simulink model "STR_Test_Template_2024_Abgabe"  (R2024a)
settings: Solver=FixedStepDiscrete  StartTime=0.0  StopTime=inf  FixedStep=.01  RelTol=1e-3  EnableMultiTasking=on
libraries: simulink x5
Description:
  | Provides a STR algorithm with variable
  | control structure, depending on the zeros of Zc
  | 
  | Order to switch on:
  | 1. Estimater
  | 2. Design
  | 3. Controller
settings Model: Creator=jreuter  LastModifiedBy=danie
settings SolverCC: AlgebraicLoopSolver=TrustRegion
settings DataIOCC: LimitDataPoints=on  SaveFormat=Array  SignalLoggingSaveFormat=ModelDataLogs  ReturnWorkspaceOutputs=off
settings OptimizationCC: BlockReduction=off  OptimizeBlockIOStorage=off  BufferReuse=off  GlobalBufferReuse=off  ExpressionFolding=off  ExpressionDepthLimit=2147483647  LocalBlockOutputs=off  LifeSpan=inf
settings DebuggingCC: UnderspecifiedInitializationDetection=Classic  MergeDetectMultiDrivingBlocksExec=none  SolverPrmCheckMsg=warning  FcnCallInpInsideContextMsg=warning  UnconnectedInputMsg=warning  UnconnectedOutputMsg=warning  UnconnectedLineMsg=warning  StateNameClashWarn=warning  SFUnexpectedBacktrackingDiag=warning  SFNoUnconditionalDefaultTransitionDiag=warning  SFExecutionAtInitializationDiag=none  ArithmeticOperatorsInVariantConditions=warning
settings HardwareCC: ProdBitPerPointer=32  ProdBitPerSizeT=32  ProdBitPerPtrDiffT=32  ProdLargestAtomicFloat=None  ProdIntDivRoundTo=Undefined  ProdEndianess=Unspecified  ProdWordSize=32  ProdHWDeviceType=32-bit Generic
settings ModelReferenceCC: EnableRefExpFcnMdlSchedulingChecks=on  PropagateSignalLabelsOutOfModel=off
settings SFSimCC: SimUseLocalCustomCode=off  CustomCodeUndefinedFunction=UseInterfaceOnly
settings RTWCC: Description=Generic Real-Time Target with dynamic memory allocation  SystemTargetFile=grt_malloc.tlc  TemplateMakefile=grt_malloc_default_tmf  GenerateReport=on  RTWUseLocalCustomCode=off  LaunchReport=on  GPUComputeCapability=3.5  DLArmComputeVersion=19.05
settings CodeAppCC: StateflowObjectComments=on
settings GRTTargetCC: TargetLangStandard=C89/C90 (ANSI)  CombineOutputUpdateFcns=off  GRTInterface=on  UseMalloc=on  ExtModeMexFile=noextcomm
settings ConfigComp: CovMetricSettings=dw  CovSaveCumulativeToWorkspaceVar=on  CovSaveSingleToWorkspaceVar=on  CovExternalEMLEnable=off

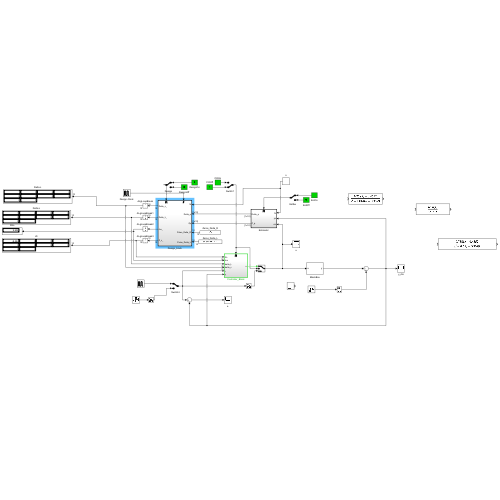
[thumbnail: Simulink's stored preview of the top-level diagram]
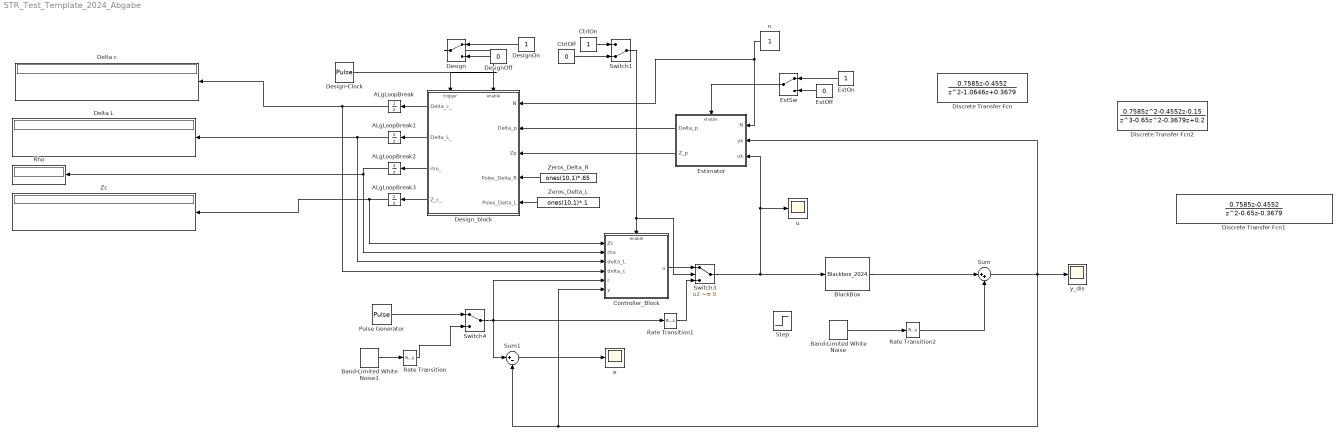
== system STR_Test_Template_2024_Abgabe ==
  ALgLoopBreak{,1..3} (4 alike) : UnitDelay  SampleTime=-1  HasFrameUpgradeWarning=on
  Band-Limited White Noise : simulink/Sources/Band-Limited White Noise  Cov=[1e-6]  Ts=.01  seed=[23341]
  Band-Limited White Noise1 : simulink/Sources/Band-Limited White Noise  Cov=[0.5]  Ts=.05  seed=[23341]
  BlackBox : S-Function  FunctionName=Blackbox_2024  SFunctionDeploymentMode=off  EnableBusSupport=off
      mask Display:
      | port_label('input',1,'u')
      | port_label('output',1,'y')
  Controller_Block : Subsystem
  CtrlOff : Constant  Value=0  SampleTime=-1
  CtrlOn : Constant  SampleTime=-1
  Delta L : Display
  Delta c : Display
  Design : ManualSwitch
  Design-Clock : DiscretePulseGenerator  PulseType=Time based  Period=.5  PulseWidth=50
  DesignOff : Constant  Value=0  SampleTime=-1
  DesignOn : Constant  SampleTime=-1
  Design_block : Subsystem
  Discrete Transfer Fcn : DiscreteTransferFcn  Numerator=[0.7585 -0.4552]  Denominator=[1 -1.0646 0.3679]
  Discrete Transfer Fcn1 : DiscreteTransferFcn  Numerator=[0.7585 -0.4552]  Denominator=[1 -0.65 -0.3679]
  Discrete Transfer Fcn2 : DiscreteTransferFcn  Numerator=[0.7585 -0.4552 -0.15]  Denominator=[1 -0.65 -0.3679 0.2]
  EstOff : Constant  Value=0  SampleTime=-1
  EstOn : Constant  SampleTime=-1
  EstSw : ManualSwitch
  Estimator : Subsystem
  Pulse Generator : DiscretePulseGenerator  PulseType=Time based  Period=1  PulseWidth=50
  Rate Transition : RateTransition  Integrity=off  OutPortSampleTimeOpt=Inherit
  Rate Transition1 : RateTransition  Integrity=off  OutPortSampleTimeOpt=Inherit
  Rate Transition2 : RateTransition  Integrity=off  OutPortSampleTimeOpt=Inherit
  Rho : Display
  Step : Step  SampleTime=0
  Sum : Sum  Inputs=|++
  Sum1 : Sum  Inputs=|+-
  Switch1 : ManualSwitch  CurrentSetting=0
  Switch3 : Switch  Criteria=u2 ~= 0  SaturateOnIntegerOverflow=off  InputSameDT=off
  Switch4 : ManualSwitch
  Zc : Display
  Zeros_Delta_L : Constant  Value=ones(10,1)*.1
  Zeros_Delta_R : Constant  Value=ones(10,1)*.65
  e : Scope
  n : Constant
  u : Scope
  y_dis : Scope
  wires:
  Band-Limited White Noise1/1 -> Rate Transition/1
  Sum/1 -> y_dis/1, Estimator/2(yk), Controller_Block/6(y), Sum1/2
  n/1 -> Estimator/1(N), Design_block/1(N)
  EstOff/1 -> EstSw/2
  EstOn/1 -> EstSw/1
  Switch1/1 -> Controller_Block/Enable, Switch3/2
  CtrlOff/1 -> Switch1/2
  CtrlOn/1 -> Switch1/1
  Estimator/1(Delta_p) -> Design_block/2(Delta_p)
  Estimator/2(Z_p) -> Design_block/3(Zp)
  Zeros_Delta_R/1 -> Design_block/4(Poles_Delta_R)
  Zeros_Delta_L/1 -> Design_block/5(Poles_Delta_L)
  Band-Limited White Noise/1 -> Rate Transition2/1
  Switch4/1 -> Rate Transition1/1, Controller_Block/5(r), Sum1/1
  Pulse Generator/1 -> Switch4/1
  Controller_Block/1(u) -> Switch3/1
  Rate Transition/1 -> Switch4/2
  Rate Transition1/1 -> Switch3/3
  Switch3/1 -> BlackBox/1, u/1, Estimator/3(uk)
  Sum1/1 -> e/1
  Design_block/4(Z_c_) -> ALgLoopBreak3/1
  Design_block/1(Delta_c_) -> ALgLoopBreak/1
  Design_block/3(rho_) -> ALgLoopBreak2/1
  Design_block/2(Delta_L_) -> ALgLoopBreak1/1
  EstSw/1 -> Estimator/Enable
  DesignOff/1 -> Design/2
  DesignOn/1 -> Design/1
  Design/1 -> Design_block/Enable
  Design-Clock/1 -> Design_block/Trigger
  ALgLoopBreak1/1 -> Delta L/1, Controller_Block/3(delta_L)
  ALgLoopBreak/1 -> Delta c/1, Controller_Block/4(delta_c)
  ALgLoopBreak3/1 -> Controller_Block/1(Zc), Zc/1
  ALgLoopBreak2/1 -> Rho/1, Controller_Block/2(rho)
  BlackBox/1 -> Sum/1
  Rate Transition2/1 -> Sum/2

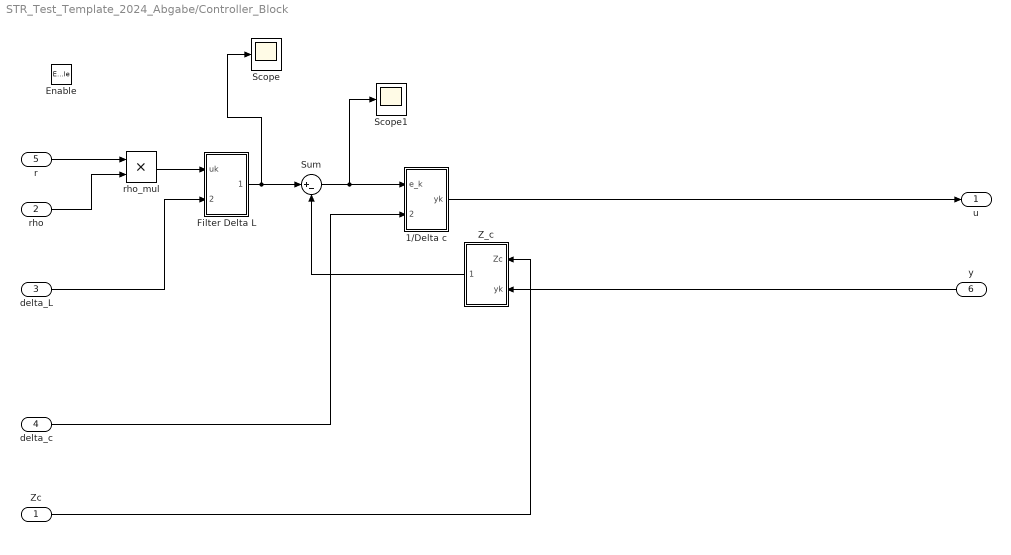
== system STR_Test_Template_2024_Abgabe/Controller_Block ==
  Zc : Inport
  rho : Inport  Port=2
  delta_L : Inport  Port=3
  delta_c : Inport  Port=4
  r : Inport  Port=5
  y : Inport  Port=6
  Enable : EnablePort  StatesWhenEnabling=reset
  1/Delta c : Subsystem
  Filter Delta L : Subsystem
  Scope : Scope
  Scope1 : Scope
  Sum : Sum  Inputs=|+-
  Z_c : Subsystem
  rho_mul : Product  RndMeth=Zero
  u : Outport
  wires:
  r/1 -> rho_mul/1
  delta_c/1 -> 1/Delta c/2(Delta_c)
  rho/1 -> rho_mul/2
  y/1 -> Z_c/2(yk)
  Sum/1 -> Scope1/1, 1/Delta c/1(e_k)
  Z_c/1(u_star) -> Sum/2
  Zc/1 -> Z_c/1(Zc)
  Filter Delta L/1(r_filtered) -> Scope/1, Sum/1
  delta_L/1 -> Filter Delta L/2(Delta_L)
  rho_mul/1 -> Filter Delta L/1(uk)
  1/Delta c/1(yk) -> u/1

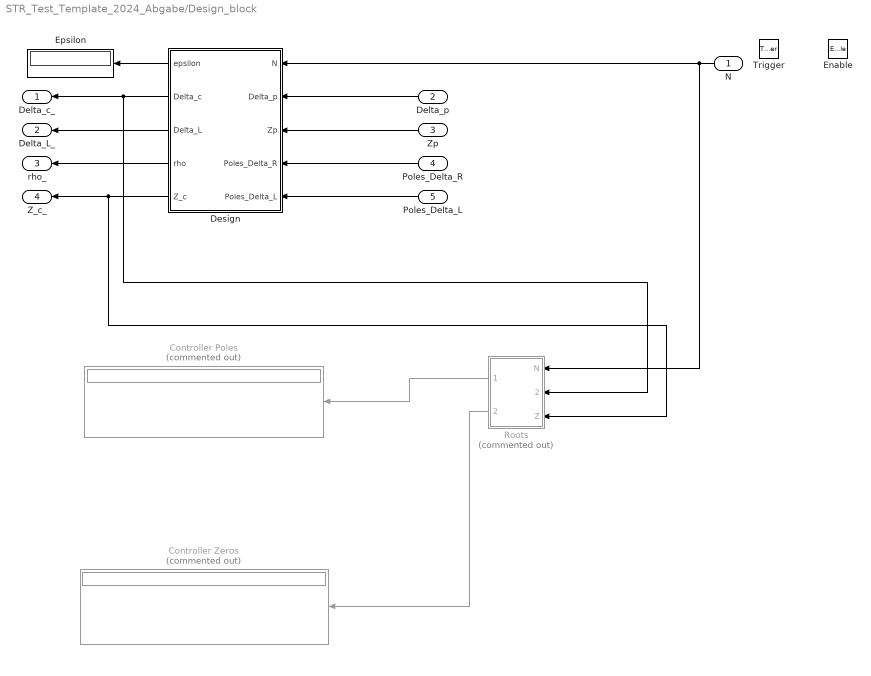
== system STR_Test_Template_2024_Abgabe/Design_block ==
  N : Inport
  Delta_p : Inport  Port=2
  Zp : Inport  Port=3
  Poles_Delta_R : Inport  Port=4
  Poles_Delta_L : Inport  Port=5
  Enable : EnablePort  StatesWhenEnabling=reset
  Trigger : TriggerPort  VariantControl=(inherit)  PortDimensions=1
  Controller Poles : Display  Commented=on
  Controller Zeros : Display  Commented=on
  Design : MATLAB Function  TreatAsAtomicUnit=on
  Epsilon : Display
  Roots : MATLAB Function  Commented=on  TreatAsAtomicUnit=on
  Delta_c_ : Outport
  Delta_L_ : Outport  Port=2
  rho_ : Outport  Port=3
  Z_c_ : Outport  Port=4
  wires:
  Design/1(epsilon) -> Epsilon/1
  N/1 -> Design/1(N), Roots/1(N)
  Delta_p/1 -> Design/2(Delta_p)
  Design/2(Delta_c) -> Delta_c_/1, Roots/2(Delta)
  Zp/1 -> Design/3(Zp)
  Design/3(Delta_L) -> Delta_L_/1
  Poles_Delta_R/1 -> Design/4(Poles_Delta_R)
  Design/4(rho) -> rho_/1
  Poles_Delta_L/1 -> Design/5(Poles_Delta_L)
  Design/5(Z_c) -> Z_c_/1, Roots/3(Z)
  Roots/1(Poles) -> Controller Poles/1
  Roots/2(Zeros) -> Controller Zeros/1

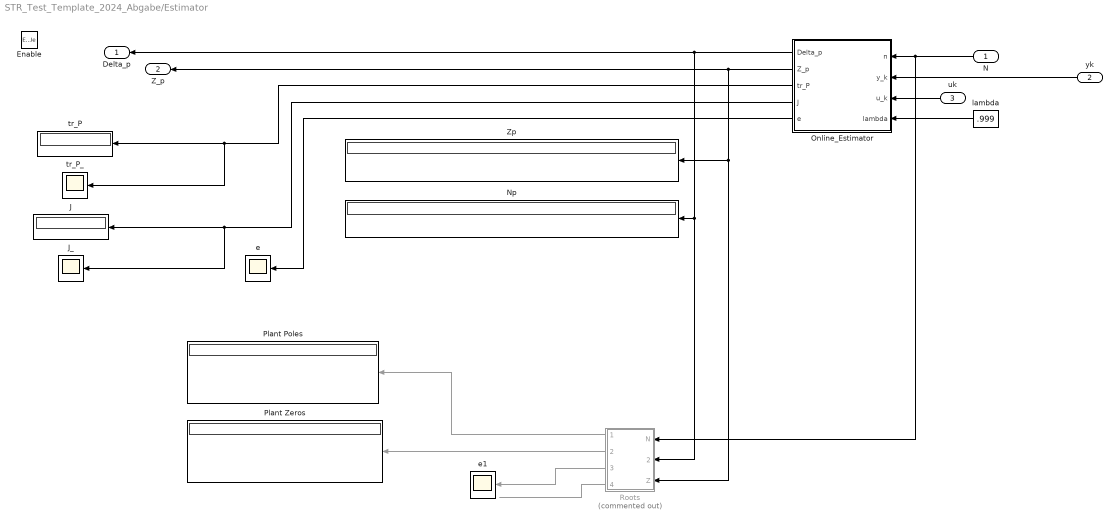
== system STR_Test_Template_2024_Abgabe/Estimator ==
  N : Inport
  yk : Inport  Port=2
  uk : Inport  Port=3
  Enable : EnablePort  StatesWhenEnabling=reset
  J : Display
  J_ : Scope
  Np : Display
  Online_Estimator : MATLAB Function  TreatAsAtomicUnit=on
  Plant Poles : Display
  Plant Zeros : Display
  Roots : MATLAB Function  Commented=on  TreatAsAtomicUnit=on
  Zp : Display
  e : Scope
  e1 : Scope
  lambda : Constant  Value=.999
  tr_P : Display
  tr_P_ : Scope
  Delta_p : Outport
  Z_p : Outport  Port=2
  wires:
  Online_Estimator/4(J) -> J_/1, J/1
  Online_Estimator/5(e) -> e/1
  Online_Estimator/3(tr_P) -> tr_P_/1, tr_P/1
  Online_Estimator/2(Z_p) -> Z_p/1, Roots/3(Z), Zp/1
  Online_Estimator/1(Delta_p) -> Roots/2(Delta), Np/1, Delta_p/1
  uk/1 -> Online_Estimator/3(u_k)
  yk/1 -> Online_Estimator/2(y_k)
  N/1 -> Roots/1(N), Online_Estimator/1(n)
  lambda/1 -> Online_Estimator/4(lambda)
  Roots/1(Poles) -> Plant Poles/1
  Roots/2(Zeros) -> Plant Zeros/1
  Roots/3(Re_Poles) -> e1/1
  Roots/4(Im_Poles) -> ?

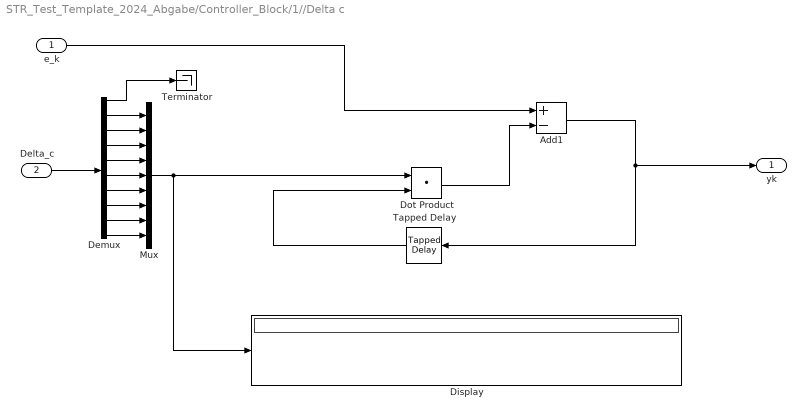
== system STR_Test_Template_2024_Abgabe/Controller_Block/1//Delta c ==
  e_k : Inport
  Delta_c : Inport  Port=2
  Add1 : Sum  Inputs=+-
  Demux : Demux  Outputs=10
  Display : Display
  Dot Product : DotProduct  OutDataTypeStr=Inherit: Inherit via internal rule
  Mux : Mux  Inputs=9
  Tapped Delay : simulink/Discrete/Tapped Delay  vinit=0.0  samptime=-1  NumDelays=9  DelayOrder=Newest  includeCurrent=off
  Terminator : Terminator
  yk : Outport
  wires:
  Tapped Delay/1 -> Dot Product/2
  Add1/1 -> Tapped Delay/1, yk/1
  e_k/1 -> Add1/1
  Dot Product/1 -> Add1/2
  Demux/10 -> Mux/9
  Demux/9 -> Mux/8
  Demux/8 -> Mux/7
  Demux/7 -> Mux/6
  Demux/6 -> Mux/5
  Demux/5 -> Mux/4
  Demux/3 -> Mux/2
  Demux/4 -> Mux/3
  Demux/2 -> Mux/1
  Delta_c/1 -> Demux/1
  Mux/1 -> Display/1, Dot Product/1
  Demux/1 -> Terminator/1

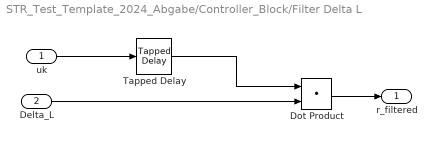
== system STR_Test_Template_2024_Abgabe/Controller_Block/Filter Delta L ==
  uk : Inport
  Delta_L : Inport  Port=2
  Dot Product : DotProduct  OutDataTypeStr=Inherit: Inherit via internal rule
  Tapped Delay : simulink/Discrete/Tapped Delay  vinit=0.0  samptime=-1  NumDelays=9  DelayOrder=Newest  includeCurrent=on
  r_filtered : Outport
  wires:
  Tapped Delay/1 -> Dot Product/1
  Dot Product/1 -> r_filtered/1
  uk/1 -> Tapped Delay/1
  Delta_L/1 -> Dot Product/2

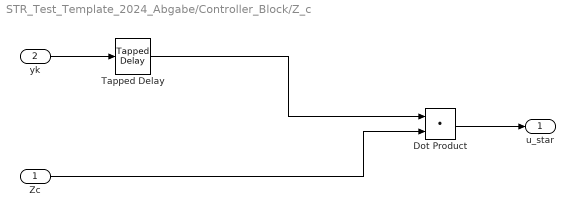
== system STR_Test_Template_2024_Abgabe/Controller_Block/Z_c ==
  Zc : Inport
  yk : Inport  Port=2
  Dot Product : DotProduct  OutDataTypeStr=Inherit: Inherit via internal rule
  Tapped Delay : simulink/Discrete/Tapped Delay  vinit=0.0  samptime=-1  NumDelays=9  DelayOrder=Newest  includeCurrent=on
  u_star : Outport
  wires:
  yk/1 -> Tapped Delay/1
  Zc/1 -> Dot Product/2
  Tapped Delay/1 -> Dot Product/1
  Dot Product/1 -> u_star/1

== matlab function STR_Test_Template_2024_Abgabe/Estimator/Online_Estimator ==
  data: Delta_p output; Z_p output; tr_P output; J output; n input; y_k input; e output; u_k input; lambda input
function [Delta_p, Z_p, tr_P, J, e  ] = fcn(n, y_k, u_k, lambda)
%eml
m = n -1;
persistent P;
persistent theta_hat;
persistent old_n; 
persistent phi;
persistent J_per;
n_max = 10;
Delta_p = zeros(1, n_max);
Z_p = zeros(1, n_max);
ek = 0;


n = min(n, n_max);

if (isempty(old_n))
    old_n = n;
end

%Initialization
if (isempty(P) || old_n ~= n) % If the order variable n has changed -> New initialization
  P = 1e4*eye(2*n_max);
  theta_hat = zeros(2*n_max, 1);
  phi = zeros(2*n_max, 1);
  old_n = n;
  J_per = 0;
end


%Your Code goes here
P = (1/lambda) * (P - ((P*phi*phi'*P)/(phi'*P*phi+lambda))); % Gewichtungsmatrix
K = (P*phi)/(phi'*P*phi+lambda);
e = y_k - phi'*theta_hat;
theta_hat = theta_hat + K*e;

% Extrahieren der vergangenen Ausgangsdaten  
phi(2:n) = phi(1:n-1);
phi(1)   = y_k;
% Extrahieren der vergangenen Eingangsdaten 
phi(n+2:n+m+1) = phi(n+1:n+m);
phi(n+1)   = u_k;
%% Ausgänge
Delta_p(1) = 1;
Delta_p(2:n+1) = theta_hat(1:n);

for i = 2:n+1
    Delta_p(i) = -Delta_p(i);
end
%Delta_p(2:n+1) = Delta_p(2:n+1) * (-1);
Z_p(1:m+1) = theta_hat(n+1:n+m+1);

tr_P = 8;
J = 0.5 * (e^2 + lambda * J_per);
J_per = J;
%J = 0;
%e = 0;

== matlab function STR_Test_Template_2024_Abgabe/Design_block/Design ==
  data: epsilon output; Delta_c output; Delta_L output; N input; Delta_p input; Zp input; rho output; Poles_Delta_R input; Z_c output; Poles_Delta_L input
function [epsilon,Delta_c ,Delta_L, rho, Z_c  ] = fcn(N, Delta_p, Zp, Poles_Delta_R, Poles_Delta_L)
%% Statische Initialisieren 
% Es werden alle Variablen statisch initialisiert um eine 
% dynamische Speicherallokation zu verhindern
n = N;
m = n-1;
max = 10; % Maximale größe

% P initial mit 0 definieren
P = zeros(max,max);
% Initialisieren von lambda und gamma mit max Length
lambda = zeros(1,max); % Initialisieren mit maxLength
gamma  = zeros(1,max); % Initialisieren mit maxLength
% Matrizen für Pseudoinverse vordefinieren
U = zeros(max,max);
S = zeros(max,max);
V = zeros(max,max);

Delta_c = zeros(max,1);
Z_c     = zeros(max,1);
Delta_L = zeros(max,1);

len_deltaP = n+1;
len_Zp     = m+1;

%% Besimmung von n und m und den Koeffizenten von delta_R und delta_L
coeffs_delta_R = poly(Poles_Delta_R(1:n));
coeffs_delta_L = poly(Poles_Delta_L(1:m));

%% Bestimmung der Vektoren Gamma und Lambda
x = conv(coeffs_delta_R, coeffs_delta_L);
gamma(1:length(x)-1) = x(2:end);
gamma = transpose(gamma);
start_index = min(len_deltaP - 1, n); 
lambda(1:start_index) = Delta_p(2:start_index+1);
lambda = transpose(lambda);

%% Erstellung der Matrix P + Invertieren durch Pseudoinverse
P = create_P(Delta_p,Zp,n,m,P,len_Zp,len_deltaP)
% Singulärwertzerlegung (SVD)
[U, S, V] = svd(P);
% Anzahl der Vektoren auswählen
cV = 2*m+1; 
% Pseudoinverse berechnen, indem nur die ersten n Vektoren verwendet werden
Pseudoinverse = V(:, 1:cV) * pinv(S(1:cV, 1:cV)) * U(:, 1:cV)';

%% Berechnen der Koeffizienten durch inv(P) * [gamma - lambda]
coeff = transpose(Pseudoinverse * (gamma-lambda));

%% Bestimmung delta_c, delta_l und Zc  
Delta_c(1)   = 1;
Delta_c(2:m+1) = coeff(1:m); 
Delta_L(1:length(coeffs_delta_L)) = coeffs_delta_L';

Z_c(1:length(coeff)-m)     = coeff(m+1:end); 
%% Bestimme Rho durch Vorgabe von T(1) = 1 mit z = 1

val_delta_c = polyval(flip(Delta_c),1);
val_Zp      = polyval(Zp,1);

%rho = val_Zp / val_delta_c
if val_Zp == 0
    rho = 1;
else
    rho = polyval(coeffs_delta_R,1) / val_Zp;
end    

%rho = 0.5;

%% Bestimmung von epsilon :: TODO
leftSide  = polyval(conv(coeffs_delta_R, coeffs_delta_L),1);
rightSide = polyval(conv(Delta_c,Delta_p),1) + polyval(conv(Zp,Z_c),1);

epsilon = leftSide - rightSide;

end
%% Funktionen 
function P = create_P(Delta_p,Zp,n,m,P, len_Zp, len_deltaP)
    % Erstellung p1_p_delta Dimension (m x m) untere Rechte Dreiecksmatrix
    % (1,1)(1,m)
    % (m,1)(m,m) 
    for i = 1:m
        P(i,1:i) = Delta_p(i:-1:1);
    end
    % Erstellung p2_p_delta Dimension (n x m)
    % (m+1  ,1)(m+1   ,m) 
    % (m+n+1,1)(m+n+1 ,m) 
    % 1. Zeile der Matrix p1 bis p(n-1)
    index = len_deltaP -1;
    for j = 1:m 
        P(m+1,j) = Delta_p(index);
        index = index -1;
    end
    % Obere Rechte Dreieckmatrix erstellen ab Zeile 2
    cStart = 1;
    for i = m+2:2*m+1
        index = len_deltaP;
        for j = cStart:m
            P(i,j) = Delta_p(index);
            index = index - 1;
        end
        cStart = cStart +1;
    end
    % Erstellung p1_c_pi Dimension (n x m)
    % (1 ,m+1)(1 ,2m+2) 
    % (m ,m+1)(m ,2m+2) 
    z = 1;
    count = 0;
    for i = m:-1:1 % Schleife Rückwärtsdurchlaufen
        for j = m+1:2*m+1
            index = len_Zp -z;
            if index <= 0
                break; % Index außerhalb der gültigen Bereichs -> 0 auffüllen
            end
            P(i,j) = Zp(index);
            z = z + 1;
        end
        count = count +1;
        z = 1 + count;
    end
    % Erstellung p2_c_pi Dimension (n x m)
    % (m+1  ,m+1)(m+1 ,2m+1) 
    % (m+n  ,m+1)(m+n ,2m+1)
    for i = m+1:m+n
        index = len_Zp;
        for j = i:2*m+1
            if index > 0
                P(i,j) = Zp(index);
                index = index - 1;
            else
                break; % Da index <= 0, kann die Schleife beenden
            end
        end
    end
end

== matlab function STR_Test_Template_2024_Abgabe/Design_block/Roots ==
  data: Poles output; Zeros output; N input; Delta input; Z input
function [Poles, Zeros  ] = fcn(N, Delta, Z)
%eml 

n_max = 10;
Poles= 1i*zeros(n_max,1);
Zeros = 1i*zeros(n_max,1);


n = min(N, n_max);
% Convert roots to coefs
Poles(1:n-1) = roots(Delta(1:n));
Zeros(1:n-1) = roots(Z(1:n));

== matlab function STR_Test_Template_2024_Abgabe/Estimator/Roots ==
  data: Poles output; Zeros output; N input; Delta input; Z input; Re_Poles output; Im_Poles output
function [Poles, Zeros, Re_Poles, Im_Poles   ] = fcn(N, Delta, Z)
%eml 

n_max = 10;
Poles= 1i*zeros(n_max,1);
Zeros = 1i*zeros(n_max,1);


n = min(N, n_max);
% Convert roots to coefs
Poles(1:n) = roots(Delta(1:n+1));
if (sum(abs(Z)) ~= 0 )
  Zeros(1:n-1) = roots(Z(2:n+1));
end

Re_Poles = real(Poles); 
Im_Poles = imag(Poles);
